simulink model "Galvo_compare_cc_and_nocc_SUB_cc_v1"  (R2013a)
settings: Solver=ode45  StartTime=0.0  StopTime=5e-3  MaxStep=1e-4  RelTol=1e-3  AbsTol=1e-5
PreLoadFcn:
  | vname=@(x) inputname(1);
  | paramCtrl=evalin('base','paramCtrl;');
  | I_LIM=str2num(paramCtrl.I_LIM);
  | Kbc=str2num(paramCtrl.Kbc);
InitFcn:
  | I_LIM=str2num(paramCtrl.I_LIM);
  | Kbc=str2num(paramCtrl.Kbc);
StartFcn:
  | I_LIM=str2num(paramCtrl.I_LIM);
  | Kbc=str2num(paramCtrl.Kbc);
values from neighbouring files (symbols this model uses):
  Lc = 170e-6    (= 0.00017)    [GalvoModel_v6_sys.m]    (also in Galvo_process_analyze.m)
  Rc = 1.5    [GalvoModel_v6_sys.m]    (also in Galvo_process_analyze.m; frequenzgang_nichtinvert_opamp_koblitz_eas.m = 1)
  Rsh = 0.003    [GalvoModel_v6_sys.m]    (also in Galvo_sys_proto_v13_OFFSETS_MODEL_PT1B_proc.m = 0.075; frequenzgang_nichtinvert_opamp_koblitz_eas.m = 0.015)
undefined symbols (not defined in the file or in its folder): JR, KBM, KFR, KMT, KTB
libraries: simulink x2
settings Model: BufferReuse=off  Creator=mainster  LastModifiedBy=mainster
settings OptimizationCC: BlockReduction=off  OptimizeBlockIOStorage=off  BufferReuse=off  ExpressionFolding=off  LocalBlockOutputs=off
settings ModelReferenceCC: ModelReferenceNumInstancesAllowed=Single

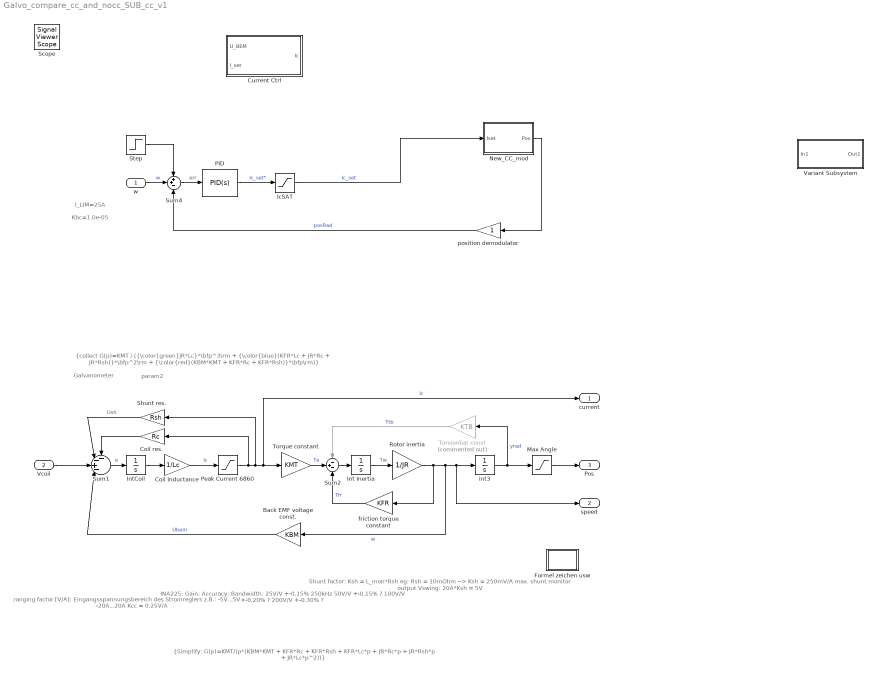
== system Galvo_compare_cc_and_nocc_SUB_cc_v1 ==
  note: I_LIM=25A
  note: Kbc=1.0e-05
  note: {Simplify: G(p)=KMT/(p*(KBM*KMT + KFR*Rc + KFR*Rsh + KFR*Lc*p + JR*Rc*p + JR*Rsh*p + JR*Lc*p^2))}
  note: {collect G(p)=KMT / ({\color{green}JR*Lc}*\bfp^3\rm + {\color{blue}(KFR*Lc + JR*Rc + JR*Rsh)}*\bfp^2\rm + {\color{red}(KBM*KMT + KFR*Rc + KFR*Rsh)}*\bfp\rm)}
  note: param2
  note: Galvanometer
  note: ranging factor [V/A]:
      | Eingangsspannungsbereich des
      | Stromreglers z.B.:
      | -5V...5V --> -20A...20A
      | Kcc = 0.25V/A
  note: Shunt factor:
      | Ksh = L_mon*Rsh
      |
      | eg: Rsh = 10mOhm
      |
      | --> Ksh = 250mV/A
      | max. shunt monitor
      | output Vswing:
      | 20A*Ksh = 5V
  note: INA225:
      | Gain:		Accuracy:		Bandwidth:
      | 25V/V		+-0.15%		250kHz
      | 50V/V		+-0.15%		?
      | 100V/V	+-0.20%		?
      | 200V/V	+-0.30%		?
  w : Inport
  Vcoil : Inport  Port=2
  Back EMF voltage const. : Gain  Gain=KBM
  Coil Inductance : Gain  Gain=1/Lc
  Coil res. : Gain  Gain=Rc
  Current Ctrl : Subsystem
  Formel zeichen usw : Subsystem
  IcSAT : Saturate  UpperLimit=I_LIM  LowerLimit=-I_LIM
  Int Inertia : Integrator
  IntCoil : Integrator
  Max Angle : Saturate  UpperLimit=20*pi/180  LowerLimit=-20*pi/180
      settings: AttributesFormatString=Max=%<UpperLimit>\nMin=%<LowerLimit>
  New_CC_mod : Subsystem
  PID : simulink/Continuous/PID Controller  Controller=PID  TimeDomain=Continuous-time  SampleTime=1  IntegratorMethod=Forward Euler  FilterMethod=Forward Euler  Form=Ideal  P=0.582255500970855  I=10.299809554028  D=0.0214479671199487  N=4765.93232634932  InitialConditionSource=internal  InitialConditionForIntegrator=0  InitialConditionForFilter=0  ExternalReset=none  IgnoreLimit=on  LimitOutput=on  UpperSaturationLimit=I_LIM  LowerSaturationLimit=-I_LIM  LinearizeAsGain=off  AntiWindupMode=back-calculation  Kb=0.01  TrackingMode=off  Kt=0  PParamMin=[]  PParamMax=[]  IParamMin=[]  IParamMax=[]  DParamMin=[]  DParamMax=[]  NParamMin=[]  NParamMax=[]  KbParamMin=[]  KbParamMax=[]  KtParamMin=[]  KtParamMax=[]  POutMin=[]  POutMax=[]  IOutMin=[]  IOutMax=[]  DOutMin=[]  DOutMax=[]  NOutMin=[]  NOutMax=[]  KbOutMin=[]  KbOutMax=[]  KtOutMin=[]  KtOutMax=[]  IntegratorOutMin=[]  IntegratorOutMax=[]  FilterOutMin=[]  FilterOutMax=[]  SumOutMin=[]  SumOutMax=[]  SumI1OutMin=[]  SumI1OutMax=[]  SumI2OutMin=[]  SumI2OutMax=[]  SumI3OutMin=[]  SumI3OutMax=[]  SumDOutMin=[]  SumDOutMax=[]  SaturationOutMin=[]  SaturationOutMax=[]  IntegratorContinuousStateAttributes=''  IntegratorStateMustResolveToSignalObject=off  IntegratorRTWStateStorageClass=Auto  FilterContinuousStateAttributes=''  FilterStateMustResolveToSignalObject=off  FilterRTWStateStorageClass=Auto
      settings: AttributesFormatString=AWM=%<AntiWindupMode>\nD=%<D>\nI=%<I>\nN=%<N>\nP=%<P>\nLimit=+-%<UpperSaturationLimit>
  Peak Current 6860 : Saturate  UpperLimit=30  LowerLimit=-30
      settings: AttributesFormatString=+-%<UpperLimit>A
  Rotor inertia : Gain  Gain=1/JR
  Shunt res. : Gain  Gain=Rsh
  Step : Step  Time=1e-3  After=10*pi/180  SampleTime=0  ZeroCross=off
      settings: AttributesFormatString=Ampl.: %<After>
  Sum1 : Sum  Inputs=--+-|
  Sum2 : Sum  Inputs=-+-
  Sum4 : Sum  Inputs=++-
  Torque constant : Gain  Gain=KMT
  Torsionbar const : Gain  Commented=on  Gain=KTB
  Variant Subsystem : Subsystem  Variant=on
  friction torque constant : Gain  Gain=KFR
  int3 : Integrator
  position demodulator : Gain
  current : Outport
  speed : Outport  Port=2
  Pos : Outport  Port=3
  Scope : SignalViewerScope  IOType=viewer  NumInputPorts=5  RefreshTime=0.035000
      settings: ShowLegends=on  TimeRange=0.005  YMin=-4~-4~-1~-8.091669250237832e-57~-4.63618497254415e-55  YMax=6~8~1~0.4~20
  wires:
  Sum4/1 -> PID/1  "err"
  Step/1 -> Sum4/1
  w/1 -> Sum4/2  "w"
  position demodulator/1 -> Sum4/3  "posRad"
  PID/1 -> IcSAT/1  "Ic_set*"
  Shunt res./1 -> Sum1/2  "Ush"
  Coil res./1 -> Sum1/1
  Vcoil/1 -> Sum1/3
  Back EMF voltage const./1 -> Sum1/4  "Ubem"
  int3/1 -> Max Angle/1, Torsionbar const/1  "yrad"
  Torque constant/1 -> Sum2/2  "Te"
  Coil Inductance/1 -> Peak Current 6860/1  "Ic"
  Torsionbar const/1 -> Sum2/1  "Ttb"
  IntCoil/1 -> Coil Inductance/1
  Sum1/1 -> IntCoil/1  "e"
  Int Inertia/1 -> Rotor inertia/1  "Tw"
  Sum2/1 -> Int Inertia/1
  Rotor inertia/1 -> friction torque constant/1, speed/1, int3/1, Back EMF voltage const./1  "w"
  friction torque constant/1 -> Sum2/3  "Tfr"
  Max Angle/1 -> Pos/1
  Peak Current 6860/1 -> Shunt res./1, current/1, Torque constant/1, Coil res./1  "Ic"
  IcSAT/1 -> New_CC_mod/1(Iset)  "Ic_set"
  New_CC_mod/1(Pos) -> position demodulator/1

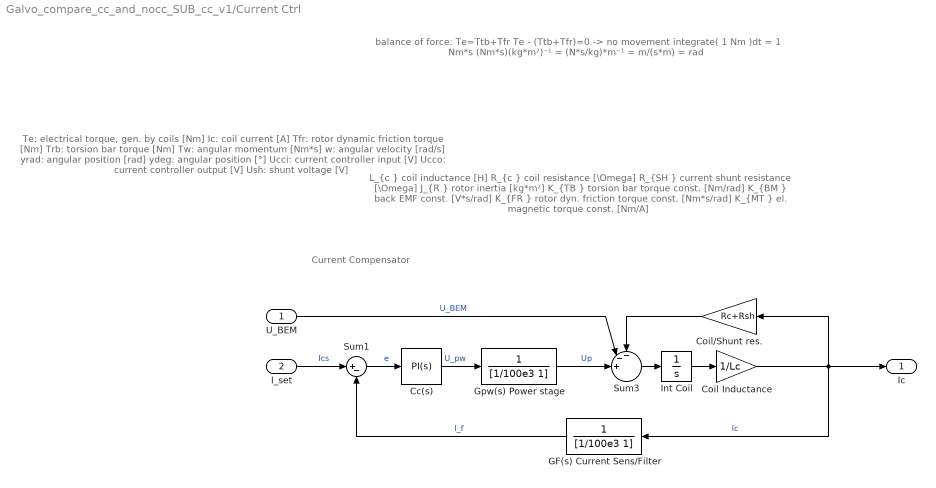
== system Galvo_compare_cc_and_nocc_SUB_cc_v1/Current Ctrl ==
  note: Current Compensator
  note: Te: 		electrical torque, gen. by coils		[Nm]
      |  Ic: 			coil current							[A]
      |  Tfr:		rotor dynamic friction torque 		[Nm]
      |  Trb:		torsion bar torque					[Nm]
      |  Tw:		angular momentum				[Nm*s]
      |  w:			angular velocity 					[rad/s]
      |  yrad:		angular position 					[rad]
      |  ydeg:		angular position 					[°]
      |  Ucci:		current controller input				[V]
      |  Ucco:		current controller output			[V]
      |  Ush:		shunt voltage						[V]
  note: L_{c  }	coil inductance 							[H]
      |  R_{c  }	coil resistance							[\Omega]
      |  R_{SH }	current shunt resistance				[\Omega]
      |  J_{R  }	rotor inertia 							[kg*m²]
      |  K_{TB }	torsion bar torque const. 			[Nm/rad]
      |  K_{BM }	back EMF const.							[V*s/rad]
      |  K_{FR }	rotor dyn. friction torque const.	[Nm*s/rad]
      |  K_{MT }	el. magnetic torque const.			[Nm/A]
  note: balance of force: 	Te=Ttb+Tfr
      | 					Te - (Ttb+Tfr)=0  ->  no movement
      |
      |  integrate( 1 Nm )dt = 1 Nm*s
      |  (Nm*s)(kg*m²)⁻¹ = (N*s/kg)*m⁻¹ = m/(s*m) = rad
  U_BEM : Inport
  I_set : Inport  Port=2
  Cc(s) : simulink/Continuous/PID Controller  Controller=PI  TimeDomain=Continuous-time  SampleTime=1  IntegratorMethod=Forward Euler  FilterMethod=Forward Euler  Form=Ideal  P=2.58986900309333  I=14540.01765706  D=0  N=100  InitialConditionSource=internal  InitialConditionForIntegrator=0  InitialConditionForFilter=0  ExternalReset=none  LimitOutput=off  UpperSaturationLimit=inf  LowerSaturationLimit=-inf  LinearizeAsGain=on  AntiWindupMode=none  Kb=1  TrackingMode=off  Kt=1  PParamMin=[]  PParamMax=[]  IParamMin=[]  IParamMax=[]  DParamMin=[]  DParamMax=[]  NParamMin=[]  NParamMax=[]  KbParamMin=[]  KbParamMax=[]  KtParamMin=[]  KtParamMax=[]  POutMin=[]  POutMax=[]  IOutMin=[]  IOutMax=[]  DOutMin=[]  DOutMax=[]  NOutMin=[]  NOutMax=[]  KbOutMin=[]  KbOutMax=[]  KtOutMin=[]  KtOutMax=[]  IntegratorOutMin=[]  IntegratorOutMax=[]  FilterOutMin=[]  FilterOutMax=[]  SumOutMin=[]  SumOutMax=[]  SumI1OutMin=[]  SumI1OutMax=[]  SumI2OutMin=[]  SumI2OutMax=[]  SumI3OutMin=[]  SumI3OutMax=[]  SumDOutMin=[]  SumDOutMax=[]  SaturationOutMin=[]  SaturationOutMax=[]  IntegratorContinuousStateAttributes=''  IntegratorStateMustResolveToSignalObject=off  IntegratorRTWStateStorageClass=Auto  FilterContinuousStateAttributes=''  FilterStateMustResolveToSignalObject=off  FilterRTWStateStorageClass=Auto
  Coil Inductance : Gain  Gain=1/Lc
  Coil/Shunt res. : Gain  Gain=Rc+Rsh
  GF(s) Current Sens/Filter : TransferFcn  Denominator=[1/100e3 1]
  Gpw(s) Power stage : TransferFcn  Denominator=[1/100e3 1]
  Int Coil : Integrator
  Sum1 : Sum  Inputs=|+-
  Sum3 : Sum  Inputs=--+||
  Ic : Outport
  wires:
  Cc(s)/1 -> Gpw(s) Power stage/1  "U_pw"
  GF(s) Current Sens/Filter/1 -> Sum1/2  "I_f"
  Coil/Shunt res./1 -> Sum3/1
  Sum3/1 -> Int Coil/1
  Gpw(s) Power stage/1 -> Sum3/3  "Up"
  Coil Inductance/1 -> Ic/1, GF(s) Current Sens/Filter/1, Coil/Shunt res./1  "Ic"
  I_set/1 -> Sum1/1  "Ics"
  Sum1/1 -> Cc(s)/1  "e"
  Int Coil/1 -> Coil Inductance/1
  U_BEM/1 -> Sum3/2  "U_BEM"

== system Galvo_compare_cc_and_nocc_SUB_cc_v1/Formel zeichen usw ==
  note: Te: 		electrical torque, gen. by coils		[Nm]
      |  Ic: 			coil current							[A]
      |  Tfr:		rotor dynamic friction torque 		[Nm]
      |  Trb:		torsion bar torque					[Nm]
      |  Tw:		angular momentum				[Nm*s]
      |  w:			angular velocity 					[rad/s]
      |  yrad:		angular position 					[rad]
      |  ydeg:		angular position 					[°]
      |  Ucci:		current controller input				[V]
      |  Ucco:		current controller output			[V]
      |  Ush:		shunt voltage						[V]
  note: L_{c  }	coil inductance 							[H]
      |  R_{c  }	coil resistance							[\Omega]
      |  R_{SH }	current shunt resistance				[\Omega]
      |  J_{R  }	rotor inertia 							[kg*m²]
      |  K_{TB }	torsion bar torque const. 			[Nm/rad]
      |  K_{BM }	back EMF const.							[V*s/rad]
      |  K_{FR }	rotor dyn. friction torque const.	[Nm*s/rad]
      |  K_{MT }	el. magnetic torque const.			[Nm/A]
  note: balance of force: 	Te=Ttb+Tfr
      | 					Te - (Ttb+Tfr)=0  ->  no movement
      |
      |  integrate( 1 Nm )dt = 1 Nm*s
      |  (Nm*s)(kg*m²)⁻¹ = (N*s/kg)*m⁻¹ = m/(s*m) = rad

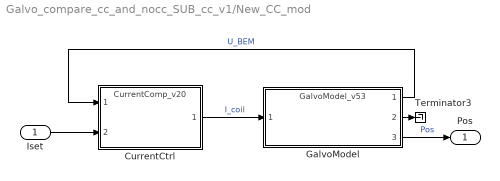
== system Galvo_compare_cc_and_nocc_SUB_cc_v1/New_CC_mod ==
  Iset : Inport
  CurrentCtrl : ModelReference  ModelNameDialog=CurrentComp_v20.slx  SimulationMode=Normal  Variant=on  OverrideUsingVariant=cc_v20  ModelReferenceVersion=1.94  CopyOfModelName=CurrentComp_v20.slx  DefaultDataLogging=on
      mask Display:
      | str=sprintf('%s',get(gcbh,'ModelName'));
      | port_label('input', 2, 'I_{Set Coil}','texmode','on')
      | color('red');
      | port_label('input', 1, 'U_{BEM}','texmode','on')
      | color('black');
      | port_label('output', 1, 'I_{Coil}','texmode','on')
      | %text(.05,.98,['{\fontsize{12}\it\bf' strrep(str,'_',' ') '}'],'horizontalAlignment','left','verticalAlignment','top','texmode','on')
      | text(.95,0.95,['{\fontsize{12}\it\bfG_{cc}(s)}'],'horizontalAlignment','right','verticalAlignment','top','texmode','on')
      | %text(.15,.05,['{\fontsize{10}\itmechanics}'],'horizontalAlignment','left','verticalAlignment','bottom','texmode','on')
  GalvoModel : ModelReference  ModelNameDialog=GalvoModel_v53.slx  SimulationMode=Normal  Variant=on  OverrideUsingVariant=v53_neuer_cc  ModelReferenceVersion=1.62  CopyOfModelName=GalvoModel_v53.slx  DefaultDataLogging=on
      mask Display:
      | str=sprintf('%s',get(gcbh,'ModelName'));
      | port_label('input', 1, 'I_{Coil}','texmode','on')
      | color('blue');
      | port_label('output', 3, 'Pos','texmode','on')
      | color('black');
      | port_label('output', 2, 'Speed','texmode','on')
      | port_label('output', 1, 'U_{BEM}','texmode','on')
      | %text(.05,.98,['{\fontsize{12}\it\bf' strrep(str,'_',' ') '}'],'horizontalAlignment','left','verticalAlignment','top','texmode','on')
      | text(.015,.98,['{\fontsize{12}\it\bf' strrep(str,'_','\_') '}'],'horizontalAlignment','left','verticalAlignment','top','texmode','on')
      | text(.15,.05,['{\fontsize{10}\itmechanics}'],'horizontalAlignment','left','verticalAlignment','bottom','texmode','on')
  Terminator3 : Terminator
  Pos : Outport
  wires:
  GalvoModel/1 -> CurrentCtrl/1  "U_BEM"
  CurrentCtrl/1 -> GalvoModel/1  "I_coil"
  Iset/1 -> CurrentCtrl/2
  GalvoModel/3 -> Pos/1  "Pos"
  GalvoModel/2 -> Terminator3/1

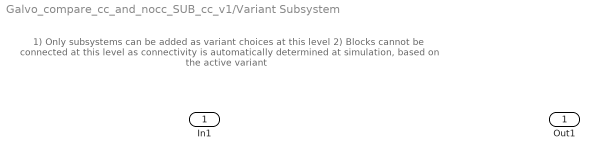
== system Galvo_compare_cc_and_nocc_SUB_cc_v1/Variant Subsystem ==
  note: 1) Only subsystems can be added as variant choices at this level
      | 2) Blocks cannot be connected at this level as connectivity is
      | automatically determined at simulation, based on the active variant
  In1 : Inport
  Out1 : Outport
